simulink model "ArduPlane_LindiPlane"  (R2018b)
settings: Solver=FixedStepDiscrete  StartTime=0.0  StopTime=1000  FixedStep=double(lindi_notune.ts)  RelTol=1e-4
libraries: simulink x3, ardupilot_custom_controller_lib x2, lindiPlane_lib x1, axes_transformation_lib x1
settings Model: DataTypeOverride=Single  DataTypeOverrideAppliesTo=Floating-point  TunableVars=lindi  TunableVarsStorageClass=Auto  Creator=Yannic  LastModifiedBy=yannic
settings SolverCC: ZeroCrossControl=DisableAll
settings DataIOCC: LimitDataPoints=on  SaveOutput=off  SaveTime=off  ReturnWorkspaceOutputs=on
settings OptimizationCC: DefaultParameterBehavior=Inlined  UseDivisionForNetSlopeComputation=on  UseFloatMulNetSlope=on  DefaultUnderspecifiedDataType=single  InlineInvariantSignals=on  PassReuseOutputArgsAs=Individual arguments  ZeroExternalMemoryAtStartup=off  ZeroInternalMemoryAtStartup=off  NoFixptDivByZeroProtection=on  EfficientFloat2IntCast=on  LifeSpan=1  OptimizeBlockOrder=speed  DifferentSizesBufferReuse=on
settings DebuggingCC: ReadBeforeWriteMsg=DisableAll  WriteAfterWriteMsg=DisableAll  WriteAfterReadMsg=DisableAll  MultiTaskDSMMsg=none  ParameterTunabilityLossMsg=error  AllowSymbolicDim=off  LibraryContextMissingDiagnostic=none  SFUnexpectedBacktrackingDiag=warning  SFNoUnconditionalDefaultTransitionDiag=warning  SFExecutionAtInitializationDiag=none
settings HardwareCC: ProdBitPerLong=64  ProdLongLongMode=on  ProdHWDeviceType=Intel->x86-64 (Linux 64)
settings ModelReferenceCC: UpdateModelReferenceTargets=IfOutOfDate  PropagateSignalLabelsOutOfModel=off
settings SFSimCC: SFSimEcho=off  SimUseLocalCustomCode=off  MATLABDynamicMemAlloc=off
settings RTWCC: SystemTargetFile=ert.tlc  GenCodeOnly=on  TemplateMakefile=ert_default_tmf  GenerateReport=on  RTWUseLocalCustomCode=off  CustomSourceCode=//custom_source_file_import_identifier  CustomHeaderCode=//custom_header_file_import_identifier  IncludeHyperlinkInReport=on  LaunchReport=on  TargetLang=C++  GenerateTraceInfo=on  GenerateTraceReport=on  GenerateTraceReportSl=on  GenerateTraceReportSf=on  GenerateTraceReportEml=on
settings CodeAppCC: ForceParamTrailComments=on  IgnoreCustomStorageClasses=off  OperatorAnnotations=on  SimulinkDataObjDesc=on  SFDataObjDesc=on  CustomSymbolStrGlobalVar=rt$N$M  CustomSymbolStrType=$N$M  CustomSymbolStrFcn=$N$M$F  CustomSymbolStrMacro=$N$M  InsertBlockDesc=on  MATLABSourceComments=on
settings ERTTargetCC: TargetLangStandard=C++03 (ISO)  IncludeMdlTerminateFcn=off  CombineSignalStateStructs=on  SuppressErrorStatus=on  SupportAbsoluteTime=off  MultiInstanceERTCode=on  CodeInterfacePackaging=C++ class  SupportNonFinite=off  SupportComplex=off  SupportVariableSizeSignals=on  ERTHeaderFileRootName=MatlabController$E  ERTSourceFileRootName=MatlabController$E  ERTDataFileRootName=MatlabController_data  InlinedParameterPlacement=NonHierarchical  RootIOFormat=Structure reference  ERTCustomFileTemplate=example_file_process.tlc  ERTFilePackagingFormat=CompactWithDataFile
settings ConfigComp: CovMetricSettings=dw  CovHtmlReporting=on  CovSaveCumulativeToWorkspaceVar=on  CovSaveSingleToWorkspaceVar=on  CovExternalEMLEnable=off

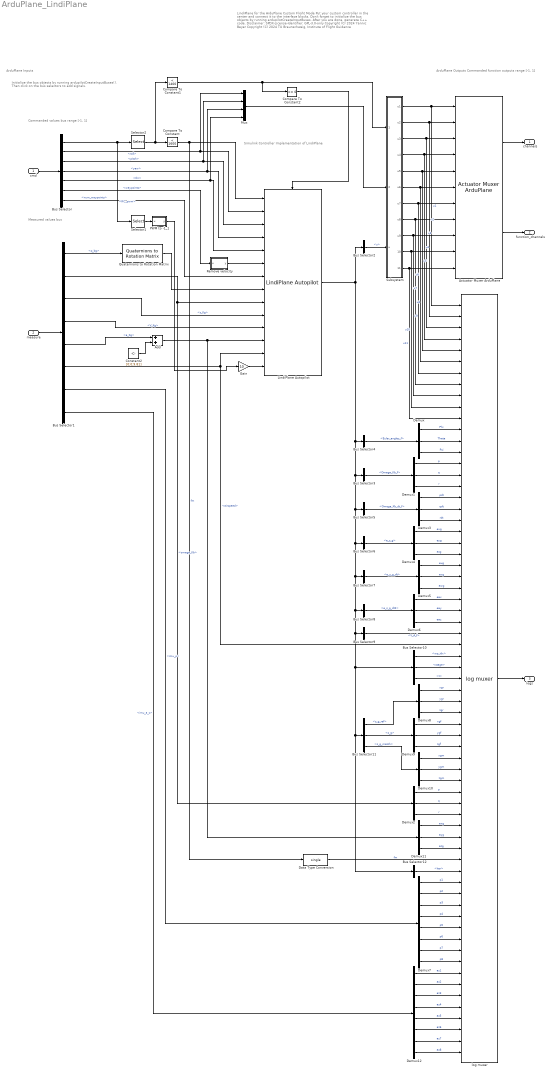
== system ArduPlane_LindiPlane ==
  note: Measured values bus
  note: Initialize the bus objects by running ardupilotCreateInputBuses().
      | Then click on the bus selectors to add signals.
  note: Commanded values bus
      | range [-1, 1]
  note: ArduPlane Inputs
  note: ArduPlane Outputs
      | Commanded function outputs
      | range [-1, 1]
  note: Simulink Controller
      | Implementation of
      | LindiPlane
  note: LindiPlane for the ArduPlane Custom Flight Mode
      |
      | Put your custom controller in the center and connect it to the interface blocks.
      | Don't forget to initialize the bus objects by running ardupilotCreateInputBuses.
      | After you are done, generate C++ code.
      |
      | Disclaimer:
      | SPDX-License-Identifier: GPL-3.0-only
      |
      | Copyright (C) 2024 Yannic Beyer
      | Copyright (C) 2024 TU Braunschweig, Institute of Flight Guidance
  cmd : Inport  OutDataTypeStr=Bus: cmdBus
  measure : Inport  Port=2  OutDataTypeStr=Bus: measureBus
  Actuator Muxer ArduPlane : ardupilot_custom_controller_lib/Actuator Muxer ArduPlane  num_channels=11  CHFCN1=passthrough  CHFCN2=passthrough  CHFCN3=passthrough  CHFCN4=passthrough  CHFCN5=passthrough  CHFCN6=passthrough  CHFCN7=passthrough  CHFCN8=passthrough  CHFCN9=k_elevator  CHFCN10=k_rudder  CHFCN11=k_throttle  CHFCN12=k_none  CHFCN13=k_none  CHFCN14=k_none  CHFCN15=k_none  CHFCN16=k_none
      settings: SourceProductName=LADAC
  Add : Sum
  Bus Selector : BusSelector  OutputSignals=RC_pwm,roll,pitch,yaw,thr,waypoints,num_waypoints
  Bus Selector1 : BusSelector  OutputSignals=q_bg,omega_Kb,s_Kg,V_Kg,a_Kg,airspeed,imu_p,imu_a_z
  Bus Selector10 : BusSelector  OutputSignals=wpnav.wp_idx,wpnav.stage,wpnav.t
  Bus Selector11 : BusSelector  OutputSignals=pos_control.reference.s_g_ref,pos_control.measure.s_g,wpnav.s_g_match
  Bus Selector12 : BusSelector  OutputSignals=inner_loop_indi.iter
  Bus Selector2 : BusSelector  OutputSignals=inner_loop_indi.u
  Bus Selector3 : BusSelector  OutputSignals=measurements.Omega_Kb_f
  Bus Selector4 : BusSelector  OutputSignals=measurements.Euler_angles_f
  Bus Selector5 : BusSelector  OutputSignals=measurements.Omega_Kb_dt_f
  Bus Selector6 : BusSelector  OutputSignals=pos_control.error.e_s_g
  Bus Selector7 : BusSelector  OutputSignals=pos_control.error.e_s_g_dt
  Bus Selector8 : BusSelector  OutputSignals=pos_control.error.e_s_g_dt2
  Bus Selector9 : BusSelector  OutputSignals=measurements.V_A_f
  Compare To Constant : simulink/Logic and Bit Operations/Compare To Constant  relop=<  const=1600  OutDataTypeStr=uint8
  Compare To Constant1 : simulink/Logic and Bit Operations/Compare To Constant  relop=<  const=1400  OutDataTypeStr=boolean
  Compare To Constant2 : simulink/Logic and Bit Operations/Compare To Constant  relop===  const=0  OutDataTypeStr=boolean
  Constant2 : Constant  Value=[0;0;9.81]  OutDataTypeStr=Inherit: Inherit via back propagation
  Data Type Conversion : DataTypeConversion  OutDataTypeStr=single
  Demux{,1..6,8..11} (11 alike) : Demux  Outputs=3
  Demux12 : Demux  Outputs=8
  Demux7 : Demux  Outputs=8
  Gain : Gain  Gain=10
  LindiPlane Autopilot : lindiPlane_lib/LindiPlane Autopilot  ap=lindi  ap_notune=lindi_notune  is_enable_checked=on  states_when_enabling=reset
  Mux : Mux
  PWM to -1_1 : MATLAB Function  TreatAsAtomicUnit=on
  Quaternions to Rotation Matrix : axes_transformation_lib/Quaternions to Rotation Matrix  SystemSampleTime=-1
      settings: SourceProductName=LADAC
  Remove velocity : MATLAB Function  TreatAsAtomicUnit=on
  Selector1 : Selector  InputPortWidth=16  IndexOptions=Index vector (dialog)  Indices=10  OutputSizes=1
  Selector2 : Selector  InputPortWidth=16  IndexOptions=Index vector (dialog)  Indices=8  OutputSizes=1
  Subsystem : Subsystem
  log muxer : ardupilot_custom_controller_lib/log muxer  batch_name_1='ML1'  num_signals_1=14  batch_name_2='ML2'  num_signals_2=14  batch_name_3='ML3'  num_signals_3=14  batch_name_4='ML4'  num_signals_4=14  batch_name_5='ML5'  num_signals_5=11
      settings: SourceProductName=LADAC
  channels : Outport
  function_channels : Outport  Port=2
  logs : Outport  Port=3
  wires:
  cmd/1 -> Bus Selector/1
  measure/1 -> Bus Selector1/1
  Bus Selector1/2 -> Demux2/1, LindiPlane Autopilot/9  "<omega_Kb>"
  Bus Selector/2 -> LindiPlane Autopilot/2, Mux/1  "<roll>"
  Bus Selector/3 -> LindiPlane Autopilot/3, Mux/2  "<pitch>"
  Bus Selector/4 -> LindiPlane Autopilot/4, Mux/3  "<yaw>"
  Bus Selector/5 -> LindiPlane Autopilot/5, Mux/4  "<thr>"
  Bus Selector1/4 -> LindiPlane Autopilot/11  "<V_Kg>"
  log muxer/1 -> logs/1
  Demux/1 -> log muxer/12  "Phi"
  Demux/2 -> log muxer/13  "Theta"
  Demux/3 -> log muxer/14  "Psi"
  Demux1/1 -> log muxer/15  "p"
  Demux1/2 -> log muxer/16  "q"
  Demux1/3 -> log muxer/17  "r"
  Demux3/1 -> log muxer/18  "pdt"
  Demux3/2 -> log muxer/19  "qdt"
  Demux3/3 -> log muxer/20  "rdt"
  Actuator Muxer ArduPlane/1 -> channels/1
  Actuator Muxer ArduPlane/2 -> function_channels/1
  Bus Selector1/1 -> Quaternions to Rotation Matrix/1  "<q_bg>"
  Quaternions to Rotation Matrix/1 -> LindiPlane Autopilot/8
  Bus Selector1/3 -> LindiPlane Autopilot/10  "<s_Kg>"
  Bus Selector1/5 -> Add/1  "<a_Kg>"
  Bus Selector1/6 -> LindiPlane Autopilot/13, log muxer/31  "<airspeed>"
  Bus Selector/6 -> Remove velocity/1(u)  "<waypoints>"
  LindiPlane Autopilot/1 -> Bus Selector2/1, Bus Selector12/1, Bus Selector11/1, Bus Selector10/1, Bus Selector9/1, Bus Selector8/1, Bus Selector7/1, Bus Selector6/1, Bus Selector5/1, Bus Selector3/1, Bus Selector4/1
  Bus Selector4/1 -> Demux/1  "<Euler_angles_f>"
  Bus Selector3/1 -> Demux1/1  "<Omega_Kb_f>"
  Bus Selector5/1 -> Demux3/1  "<Omega_Kb_dt_f>"
  Demux4/1 -> log muxer/21  "exg"
  Demux4/2 -> log muxer/22  "eyg"
  Demux4/3 -> log muxer/23  "ezg"
  Bus Selector6/1 -> Demux4/1  "<e_s_g>"
  Demux5/1 -> log muxer/24  "eug"
  Demux5/2 -> log muxer/25  "evg"
  Demux5/3 -> log muxer/26  "ewg"
  Bus Selector7/1 -> Demux5/1  "<e_s_g_dt>"
  Demux6/1 -> log muxer/27  "eax"
  Demux6/2 -> log muxer/28  "eay"
  Demux6/3 -> log muxer/29  "eaz"
  Bus Selector8/1 -> Demux6/1  "<e_s_g_dt2>"
  Bus Selector9/1 -> log muxer/30  "<V_A_f>"
  Bus Selector/1 -> Selector1/1, Selector2/1  "<RC_pwm>"
  Compare To Constant/1 -> LindiPlane Autopilot/1, Data Type Conversion/1  "fm"
  Selector2/1 -> Compare To Constant1/1, Compare To Constant/1
  Bus Selector2/1 -> Subsystem/3(u)  "<u>"
  Subsystem/11(u11) -> log muxer/11, Actuator Muxer ArduPlane/11  "u11"
  Subsystem/7(u7) -> log muxer/7, Actuator Muxer ArduPlane/7  "u7"
  Subsystem/6(u6) -> log muxer/6, Actuator Muxer ArduPlane/6  "u6"
  Subsystem/5(u5) -> log muxer/5, Actuator Muxer ArduPlane/5  "u5"
  Subsystem/3(u3) -> log muxer/3, Actuator Muxer ArduPlane/3  "u3"
  Subsystem/2(u2) -> log muxer/2, Actuator Muxer ArduPlane/2  "u2"
  Subsystem/1(u1) -> log muxer/1, Actuator Muxer ArduPlane/1  "u1"
  Subsystem/8(u8) -> log muxer/8, Actuator Muxer ArduPlane/8  "u8"
  Subsystem/9(u9) -> log muxer/9, Actuator Muxer ArduPlane/9  "u9"
  Subsystem/10(u10) -> log muxer/10, Actuator Muxer ArduPlane/10  "u10"
  Mux/1 -> Subsystem/2(rpyt)
  Compare To Constant1/1 -> Compare To Constant2/1, Subsystem/1(is_manual)
  Constant2/1 -> Add/2
  Add/1 -> Demux11/1, LindiPlane Autopilot/12
  Demux2/3 -> log muxer/46  "r"
  Demux2/2 -> log muxer/45  "q"
  Demux2/1 -> log muxer/44  "p"
  Data Type Conversion/1 -> log muxer/50  "fm"
  Bus Selector10/1 -> log muxer/32  "<wp_idx>"
  Bus Selector10/2 -> log muxer/33  "<stage>"
  Bus Selector10/3 -> log muxer/34  "<t>"
  Bus Selector11/1 -> Demux8/1  "<s_g_ref>"
  Demux8/1 -> log muxer/35  "xgr"
  Demux8/2 -> log muxer/36  "ygr"
  Demux8/3 -> log muxer/37  "zgr"
  Demux9/1 -> log muxer/38  "xgf"
  Demux9/2 -> log muxer/39  "ygf"
  Demux9/3 -> log muxer/40  "zgf"
  Bus Selector11/2 -> Demux9/1  "<s_g>"
  Demux10/1 -> log muxer/41  "xgm"
  Demux10/2 -> log muxer/42  "ygm"
  Demux10/3 -> log muxer/43  "zgm"
  Bus Selector11/3 -> Demux10/1  "<s_g_match>"
  Bus Selector/7 -> LindiPlane Autopilot/7  "<num_waypoints>"
  Demux11/3 -> log muxer/49  "azg"
  Demux11/2 -> log muxer/48  "ayg"
  Demux11/1 -> log muxer/47  "axg"
  Remove velocity/1(y) -> LindiPlane Autopilot/6
  Compare To Constant2/1 -> LindiPlane Autopilot/Enable
  Subsystem/4(u4) -> log muxer/4, Actuator Muxer ArduPlane/4  "u4"
  Bus Selector12/1 -> log muxer/51  "<iter>"
  Bus Selector1/7 -> Demux7/1  "<imu_p>"
  Bus Selector1/8 -> Demux12/1  "<imu_a_z>"
  Demux7/8 -> log muxer/59  "p8"
  Demux7/7 -> log muxer/58  "p7"
  Demux7/6 -> log muxer/57  "p6"
  Demux7/5 -> log muxer/56  "p5"
  Demux7/4 -> log muxer/55  "p4"
  Demux7/3 -> log muxer/54  "p3"
  Demux7/2 -> log muxer/53  "p2"
  Demux7/1 -> log muxer/52  "p1"
  Demux12/1 -> log muxer/60  "az1"
  Demux12/2 -> log muxer/61  "az2"
  Demux12/3 -> log muxer/62  "az3"
  Demux12/4 -> log muxer/63  "az4"
  Demux12/5 -> log muxer/64  "az5"
  Demux12/6 -> log muxer/65  "az6"
  Demux12/7 -> log muxer/66  "az7"
  Demux12/8 -> log muxer/67  "az8"
  Selector1/1 -> PWM to -1_1/1(u)
  Gain/1 -> LindiPlane Autopilot/14
  PWM to -1_1/1(y) -> Gain/1

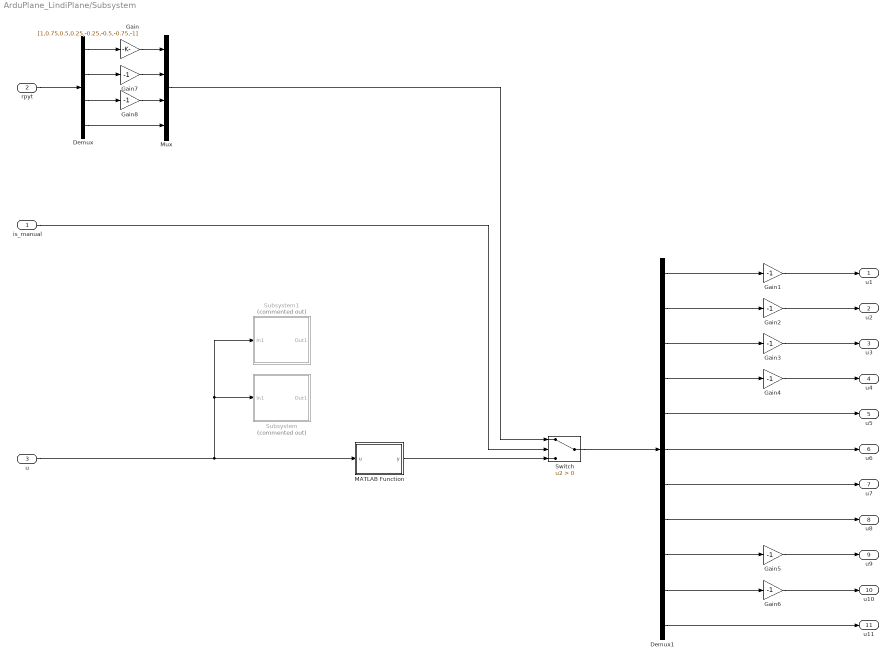
== system ArduPlane_LindiPlane/Subsystem ==
  is_manual : Inport
  rpyt : Inport  Port=2
  u : Inport  Port=3
  Demux : Demux
  Demux1 : Demux  Outputs=11
  Gain : Gain  Gain=[1,0.75,0.5,0.25,-0.25,-0.5,-0.75,-1]
  Gain{1..8} (8 alike) : Gain  Gain=-1
  MATLAB Function : MATLAB Function  TreatAsAtomicUnit=on
  Mux : Mux
  Subsystem : Subsystem  Commented=on
  Subsystem1 : Subsystem  Commented=on
  Switch : Switch  Criteria=u2 > Threshold
  u1 : Outport
  u2 : Outport  Port=2
  u3 : Outport  Port=3
  u4 : Outport  Port=4
  u5 : Outport  Port=5
  u6 : Outport  Port=6
  u7 : Outport  Port=7
  u8 : Outport  Port=8
  u9 : Outport  Port=9
  u10 : Outport  Port=10
  u11 : Outport  Port=11
  wires:
  is_manual/1 -> Switch/2
  rpyt/1 -> Demux/1
  Demux/1 -> Gain/1
  Demux/4 -> Mux/4
  Demux/3 -> Gain8/1
  Demux/2 -> Gain7/1
  Gain/1 -> Mux/1
  Mux/1 -> Switch/1
  Demux1/1 -> Gain1/1
  Demux1/2 -> Gain2/1
  Demux1/11 -> u11/1
  Demux1/10 -> Gain6/1
  Demux1/9 -> Gain5/1
  Demux1/8 -> u8/1
  Demux1/7 -> u7/1
  Demux1/6 -> u6/1
  Demux1/5 -> u5/1
  Demux1/4 -> Gain4/1
  Demux1/3 -> Gain3/1
  Gain1/1 -> u1/1
  Gain2/1 -> u2/1
  Gain3/1 -> u3/1
  Gain4/1 -> u4/1
  Switch/1 -> Demux1/1
  Gain5/1 -> u9/1
  Gain6/1 -> u10/1
  Gain7/1 -> Mux/2
  Gain8/1 -> Mux/3
  u/1 -> MATLAB Function/1(u), Subsystem1/1(In1), Subsystem/1(In1)
  MATLAB Function/1(y) -> Switch/3

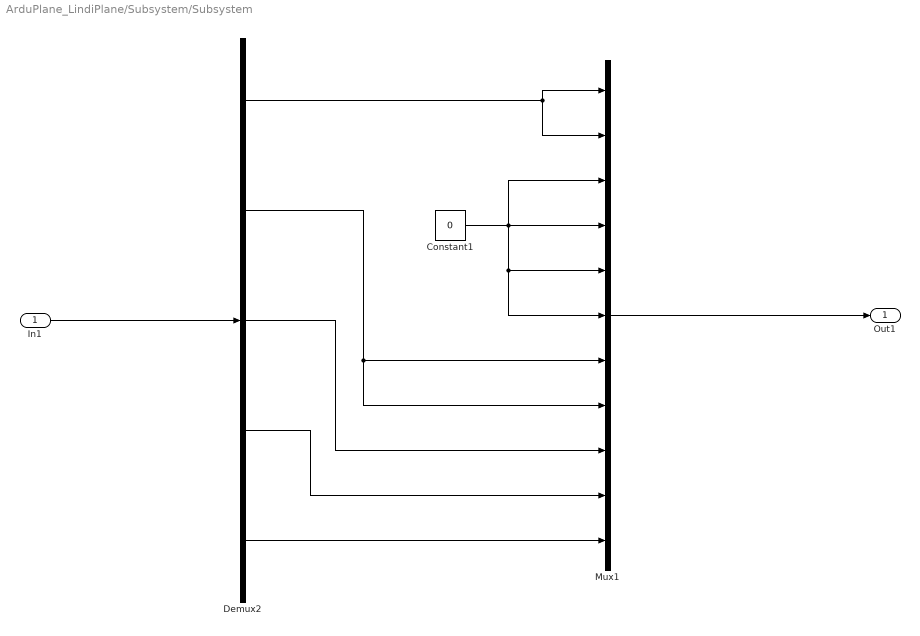
== system ArduPlane_LindiPlane/Subsystem/Subsystem ==
  In1 : Inport
  Constant1 : Constant  Value=0
  Demux2 : Demux  Outputs=5
  Mux1 : Mux  Inputs=11
  Out1 : Outport
  wires:
  Demux2/4 -> Mux1/10
  Demux2/3 -> Mux1/9
  In1/1 -> Demux2/1
  Demux2/2 -> Mux1/7, Mux1/8
  Mux1/1 -> Out1/1
  Demux2/5 -> Mux1/11
  Constant1/1 -> Mux1/3, Mux1/4, Mux1/5, Mux1/6
  Demux2/1 -> Mux1/2, Mux1/1

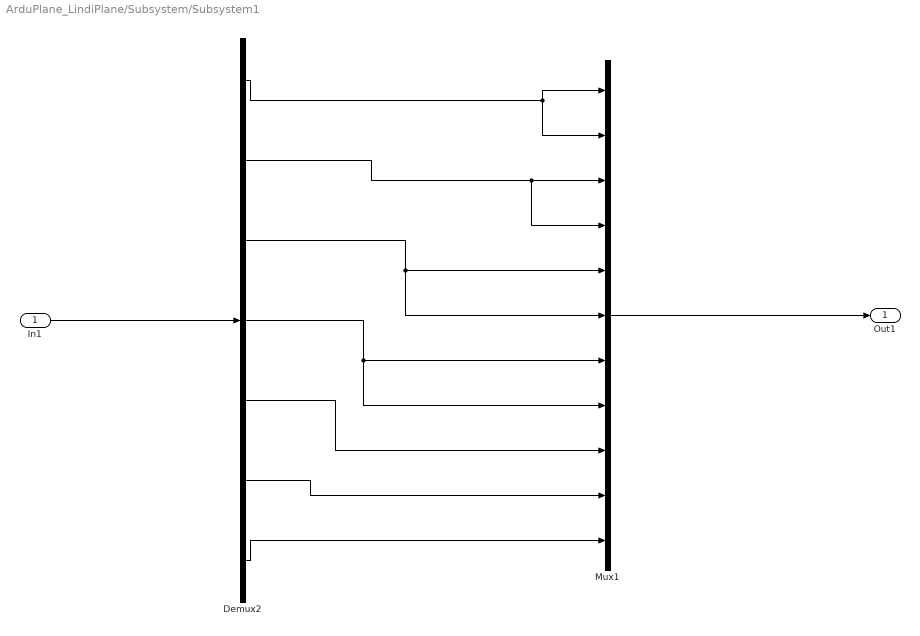
== system ArduPlane_LindiPlane/Subsystem/Subsystem1 ==
  In1 : Inport
  Demux2 : Demux  Outputs=7
  Mux1 : Mux  Inputs=11
  Out1 : Outport
  wires:
  Demux2/1 -> Mux1/1, Mux1/2
  Demux2/7 -> Mux1/11
  Mux1/1 -> Out1/1
  Demux2/4 -> Mux1/8, Mux1/7
  In1/1 -> Demux2/1
  Demux2/5 -> Mux1/9
  Demux2/6 -> Mux1/10
  Demux2/3 -> Mux1/5, Mux1/6
  Demux2/2 -> Mux1/4, Mux1/3

== matlab function ArduPlane_LindiPlane/Remove velocity ==
  data: u input; y output
function y = fcn(u)
y = u(1:3,:);
end

== matlab function ArduPlane_LindiPlane/PWM to -1_1 ==
  data: u input; y output
function y = fcn(u)
y = (u-1500)/500;
end

== matlab function ArduPlane_LindiPlane/Subsystem/MATLAB Function ==
  data: u input; y output
function y = fcn(u)
y = zeros(11,1,superiorfloat(u));
% number of flaps per wing side
num_flaps = (length(u)-3)/2;
y(1:num_flaps) = u(1:num_flaps);
y(5:4+num_flaps) = u(num_flaps+1:2*num_flaps);
y(end-2:end) = u(end-2:end);
end
